simulink model "PI_Fuzzy"  (R2017b)
settings: Solver=ode4  StartTime=0.0  StopTime=10.0  FixedStep=0.001  RelTol=1e-3
libraries: fuzblock x1
settings Model: Creator=84935  LastModifiedBy=84935

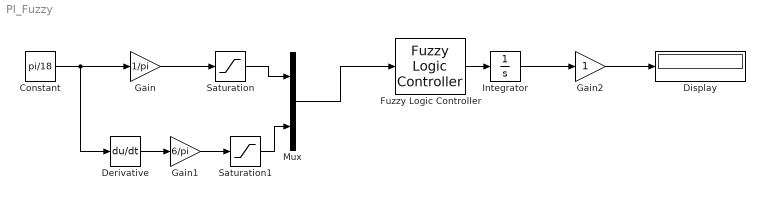
== system PI_Fuzzy ==
  Constant : Constant  Value=pi/18
  Derivative : Derivative
  Display : Display
  Fuzzy Logic Controller : fuzblock/Fuzzy Logic  Controller  FIS='PI_Fuzzy.fis'  OutputSampleNumber=101  DataType=double  FuzzifiedInputs=off  RuleFiringStrengths=off  RuleOutputs=off  AggregatedOutputs=off  SimulateUsing=Interpreted execution
  Gain : Gain  Gain=1/pi
  Gain1 : Gain  Gain=6/pi
  Gain2 : Gain
  Integrator : Integrator
  Mux : Mux  Inputs=2
  Saturation : Saturate  UpperLimit=1  LowerLimit=-1
  Saturation1 : Saturate  UpperLimit=1  LowerLimit=-1
  wires:
  Mux/1 -> Fuzzy Logic Controller/1
  Constant/1 -> Derivative/1, Gain/1
  Derivative/1 -> Gain1/1
  Fuzzy Logic Controller/1 -> Integrator/1
  Integrator/1 -> Gain2/1
  Gain2/1 -> Display/1
  Gain1/1 -> Saturation1/1
  Saturation1/1 -> Mux/2
  Gain/1 -> Saturation/1
  Saturation/1 -> Mux/1
